simulink model "symulacja_pid1w"  (R2020a)
settings: Solver=VariableStepAuto  StartTime=0.0  StopTime=10.0  RelTol=1e-3
values from neighbouring files (symbols this model uses):
  D = dec2bin(int32(m_p(:,3)*100),b_len)    [dec_bin_conv.m]    (also in funkcja_oceny.m = PID(3); funkcja_oceny_optim.m = PID(3); funkcja_oceny_wyswietlanie.m = PID(3); population_draw.m = dec2bin(D,b_len))
  I = dec2bin(int32(m_p(:,2)*100),b_len)    [dec_bin_conv.m]    (also in funkcja_oceny.m = PID(2); funkcja_oceny_optim.m = PID(2); funkcja_oceny_wyswietlanie.m = PID(2); population_draw.m = dec2bin(I,b_len))
  K = zmienne(1)    [funkcja_oceny.m]    (also in funkcja_oceny_optim.m = 3; funkcja_oceny_wyswietlanie.m; wyswietlanie_PID.m)
  P = dec2bin(int32(m_p(:,1)*100),b_len)    [dec_bin_conv.m]    (also in funkcja_oceny.m = PID(1); funkcja_oceny_optim.m = PID(1); funkcja_oceny_wyswietlanie.m = PID(1); population_draw.m = dec2bin(P,b_len))
  T1 = zmienne(3)    [funkcja_oceny.m]    (also in funkcja_oceny_optim.m = 10; funkcja_oceny_wyswietlanie.m; wyswietlanie_PID.m)
  T2 = zmienne(4)    [funkcja_oceny.m]    (also in funkcja_oceny_optim.m = 12; funkcja_oceny_wyswietlanie.m; wyswietlanie_PID.m)
  tau = zmienne(2)    [funkcja_oceny.m]    (also in funkcja_oceny_optim.m = 2; funkcja_oceny_wyswietlanie.m; wyswietlanie_PID.m)
libraries: simulink x1
settings Model: Creator=Staluga  LastModifiedBy=Staluga

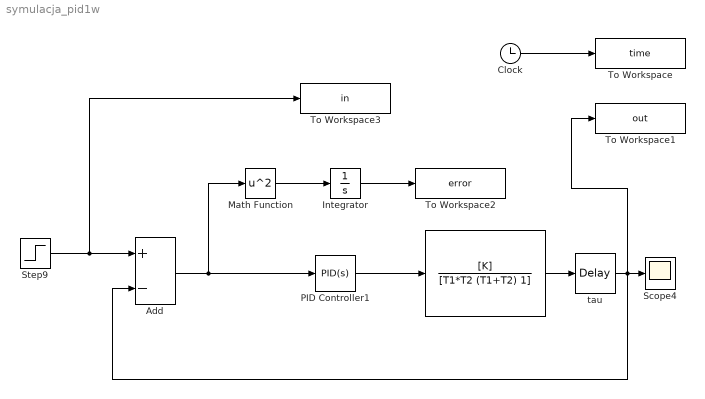
== system symulacja_pid1w ==
  " " : TransferFcn  Numerator=[K]  Denominator=[T1*T2 (T1+T2) 1]
  Add : Sum  Inputs=+-
  Clock : Clock
  Integrator : Integrator
  Math Function : Math  Operator=square  SaturateOnIntegerOverflow=on
  PID Controller1 : simulink/Continuous/PID Controller  Controller=PID  Form=Parallel  TimeDomain=Continuous-time  UseExternalTs=off  SampleTime=-1  IntegratorMethod=Forward Euler  FilterMethod=Forward Euler  ControllerParametersSource=internal  P=P  I=I  D=D  UseFilter=on  N=100  TunerSelectOption=Transfer Function Based (PID Tuner App)  InitialConditionSource=internal  InitialConditionForIntegrator=0  InitialConditionForFilter=0  DifferentiatorICPrevScaledInput=0  ExternalReset=none  TrackingMode=off  Kt=1  LimitOutput=off  UpperSaturationLimit=inf  LowerSaturationLimit=-inf  LinearizeAsGain=on  AntiWindupMode=none  Kb=1  POutMin=[]  POutMax=[]  IOutMin=[]  IOutMax=[]  DOutMin=[]  DOutMax=[]  NOutMin=[]  NOutMax=[]  SumOutMin=[]  SumOutMax=[]  SaturationOutMin=[]  SaturationOutMax=[]  PParamMin=[]  PParamMax=[]  IParamMin=[]  IParamMax=[]  DParamMin=[]  DParamMax=[]  NParamMin=[]  NParamMax=[]  KbParamMin=[]  KbParamMax=[]  KtParamMin=[]  KtParamMax=[]  KbOutMin=[]  KbOutMax=[]  KtOutMin=[]  KtOutMax=[]  IntegratorOutMin=[]  IntegratorOutMax=[]  FilterOutMin=[]  FilterOutMax=[]  SumI1OutMin=[]  SumI1OutMax=[]  SumI2OutMin=[]  SumI2OutMax=[]  SumI3OutMin=[]  SumI3OutMax=[]  SumI4OutMin=[]  SumI4OutMax=[]  SumDOutMin=[]  SumDOutMax=[]  DifferentiatorOutMin=[]  DifferentiatorOutMax=[]  FilterDiffOutCoefMin=[]  FilterDiffOutCoefMax=[]  ReciprocalOutMin=[]  ReciprocalOutMax=[]  SumDenOutMin=[]  SumDenOutMax=[]  SumNumOutMin=[]  SumNumOutMax=[]  DivideOutMin=[]  DivideOutMax=[]  UdiffTsProdOutMin=[]  UdiffTsProdOutMax=[]  NTsProdOutMin=[]  NTsProdOutMax=[]  UintegralTsProdOutMin=[]  UintegralTsProdOutMax=[]  UngainTsProdOutMin=[]  UngainTsProdOutMax=[]  IntegratorContinuousStateAttributes=''  IntegratorStateMustResolveToSignalObject=off  IntegratorRTWStateStorageClass=Auto  FilterContinuousStateAttributes=''  FilterStateMustResolveToSignalObject=off  FilterRTWStateStorageClass=Auto  ParallelPVariant=InternalParameters  IdealPVariant=Disabled  IVariant=InternalParameters  DVariant=InternalParameters  IntegratorVariant=Continuous  SatVariant=Disabled  AWVariant=Passthrough  PCopyVariant=Disabled  TRVariant=Disabled  FdbkBlocksVariant=Forward  IdealPFdbkVariant=Disabled  SatFdbkVariant=Disabled  DerivativeFilterVariant=ContFilter  NVariant=InternalParameters  NCopyVariant=Disabled  FilterICVariant=InternalICsFilter  IntegratorICVariant=InternalICs  ExternalResetVariant=Disabled  TRSumVariant=Passthrough  SumFdbkVariant=Disabled  SumVariant=Sum_PID  TsampFilterVariant=InternalTs  TsampNgainVariant=Passthrough  TsampIntegralVariant=Passthrough
  Scope4 : Scope
  Step9 : Step  SampleTime=0
  To Workspace : ToWorkspace  VariableName=time  SampleTime=-1
  To Workspace1 : ToWorkspace  VariableName=out  SampleTime=-1
  To Workspace2 : ToWorkspace  VariableName=error  SampleTime=-1
  To Workspace3 : ToWorkspace  VariableName=in  SampleTime=-1
  tau : TransportDelay  DelayTime=tau
  wires:
  Clock/1 -> To Workspace/1
  Math Function/1 -> Integrator/1
  Add/1 -> Math Function/1, PID Controller1/1
  Integrator/1 -> To Workspace2/1
  tau/1 -> To Workspace1/1, Add/2, Scope4/1
  Step9/1 -> To Workspace3/1, Add/1
  " "/1 -> tau/1
  PID Controller1/1 -> " "/1
